simulink model "Ejercicio_1_e_DB"  (R2023a)
settings: Solver=VariableStepAuto  StartTime=0.0  StopTime=10.0  RelTol=1e-3
values from neighbouring files (symbols this model uses):
  g0 = utilsMati.realim_VE.factorEscala(A,B,C,K) * 1/20    [Ejercicio_1.m]
  K = acker(A,B,PLC_VE)    [Ejercicio_1.m]
settings Model: Creator=Mati  LastModifiedBy=Mati

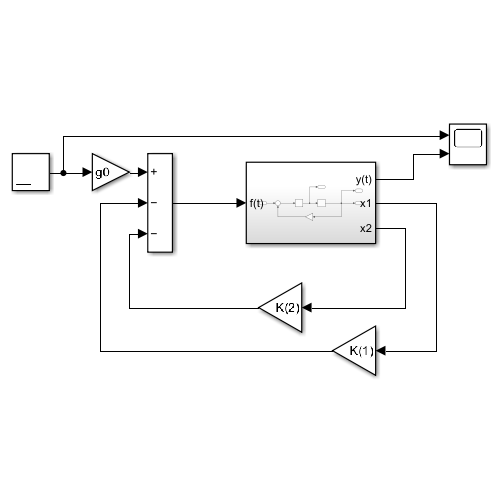
[thumbnail: Simulink's stored preview of the top-level diagram]
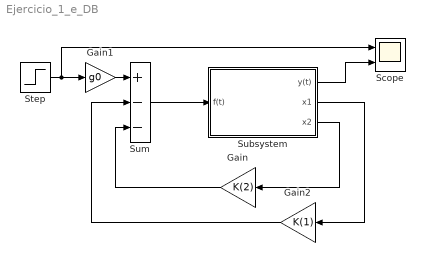
== system Ejercicio_1_e_DB ==
  Gain : Gain  Gain=K(2)
  Gain1 : Gain  Gain=g0
  Gain2 : Gain  Gain=K(1)
  Scope : Scope  NumInputPorts=2
  Step : Step  SampleTime=0
  Subsystem : Subsystem
  Sum : Sum  Inputs=+--
  wires:
  Step/1 -> Gain1/1, Scope/1
  Sum/1 -> Subsystem/1(f(t))
  Subsystem/1(y(t)) -> Scope/2
  Gain/1 -> Sum/3
  Gain2/1 -> Sum/2
  Subsystem/3(x2) -> Gain/1
  Subsystem/2(x1) -> Gain2/1
  Gain1/1 -> Sum/1

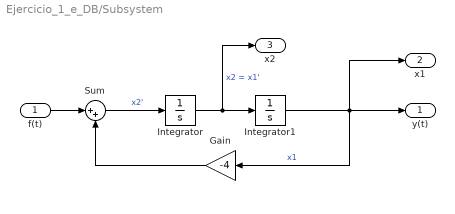
== system Ejercicio_1_e_DB/Subsystem ==
  f(t) : Inport
  Gain : Gain  Gain=-4
  Integrator : Integrator
  Integrator1 : Integrator
  Sum : Sum  Inputs=|++
  y(t) : Outport
  x1 : Outport  Port=2
  x2 : Outport  Port=3
  wires:
  f(t)/1 -> Sum/1
  Sum/1 -> Integrator/1  "x2'"
  Integrator/1 -> x2/1, Integrator1/1  "x2 = x1'"
  Integrator1/1 -> x1/1, Gain/1, y(t)/1  "x1"
  Gain/1 -> Sum/2
